simulink model "DA40_Flight_Model"  (R2023a)
settings: Solver=FixedStepAuto  StartTime=DCAM.startTime  StopTime=DCAM.endTime  FixedStep=DCAM.timeStep  RelTol=1e-3
undefined symbols (not defined in the file or in its folder): DCAM, Earth, WGS84
libraries: simulink x27, slpidlib x15, simulink_extras x6, sharedtransform x4, aerolibtransform2 x4, aerolibatmos2 x3, uavalgslib x2, aerolibwind2 x1
(part 6 of 6)

== matlab function DA40_Flight_Model/Correlator Simulation/Subsystem1/Generating GPS and Satellite Measurements1/Truth Model/Navigation1/Flight Mechanics and Systems Models/Engine + Prop Model/Subsystem/MATLAB Function ==
  data: X input; Aircraft_Airspeed output
function Aircraft_Airspeed = Calc_AC_Speed(X)
Aircraft_Airspeed = norm(X(1:3));
end

== matlab function DA40_Flight_Model/Correlator Simulation/Subsystem1/Generating GPS and Satellite Measurements1/Truth Model/Navigation1/Flight Mechanics and Systems Models/Engine + Prop Model/Subsystem/Manifold Pressure Calculation ==
  data: throttle input; Patm_inHg input; N input; Pman_inHg output; throttle output; Patm_inHg output
function [Pman_inHg,throttle,Patm_inHg]  = fcn(throttle,Patm_inHg,N)

Pman_inHg = Patm_inHg + (0.007*throttle - 0.0086)*N;

end

== matlab function DA40_Flight_Model/Correlator Simulation/Subsystem1/Generating GPS and Satellite Measurements1/Truth Model/Navigation1/Flight Mechanics and Systems Models/Engine + Prop Model/Subsystem/Propeller Dynamics ==
  data: V input; power input; Q_drive input size=1; Prop_Pitch input; rho input; n input; T output; Q output; eta_p output size=1; dOmega_dt output
function [T,Q,eta_p,dOmega_dt] = VarP_PropDynamics(V,power, Q_drive,Prop_Pitch,rho,n)

T = 0;
Q = 0;
eta_p = 0;
dOmega_dt = 0;

coder.extrinsic('griddedInterpolant')
coder.extrinsic('CTCQPropeff')

[T,Q,eta_p,dOmega_dt] = CTCQPropeff(Prop_Pitch,power,Q_drive,rho,V,n,[]);

end

== matlab function DA40_Flight_Model/Extended Kalman Filter/ECEF to BODY/MATLAB Function1 ==
  data: x output; pos input; y output; vel input; clk input; clkBias input; DCM_BL input; z output; u output; v output; w output; clk output; clkBias output; refLL input
function [x,y,z,u,v,w,clk,clkBias] = EarthToBodyStates(pos,vel,clk,clkBias,DCM_BL,refLL)
x = 0;
y = 0;
z = 0;
u = 0;
v = 0;
w = 0;

coder.extrinsic("EarthToBodyStates")

[x,y,z,u,v,w,clk,clkBias] = BodyToEarthStates(pos,vel,clk,clkBias,DCM_BL,refLL);

end

== matlab function DA40_Flight_Model/Correlator Simulation/Subsystem1/Generating GPS and Satellite Measurements1/Truth Model/Navigation1/Flight Mechanics and Systems Models/Gear/  ==
  data: U input; X input; mu input; Ground_Forces output; Ground_Moments output
function [Ground_Forces,Ground_Moments] = LDG_Model(U,X,mu)
%% Ground Contact points taken from powerpoint
Front_LDG = [1.634;0;0.983]';
Right_MG = [-0.5;1.447;0.893]';
Left_MG = [-0.5;-1.447;0.893]';
Prop_Strike = [2.379;0;0.847]';
Right_Wing = [0;5.53;-0.087]';
Left_Wing = [0;-5.53;-0.087]';
Tail_Strike = [-4.552;0;0.271]';
GC = [Front_LDG;Right_MG;Left_MG;Prop_Strike;Right_Wing;Left_Wing;Tail_Strike];
%% Spring and Damper Coeffs
k_r = 80000;
c_r = 14300;

k_f = 50000;
c_f = 11300;

k_b = 280000;
c_b = 26800;
%% Defining State Vector to make the coding easier
u = X(1);
v = X(2);
w = X(3);
p = X(4);
q = X(5);
r = X(6);
x = X(7);
y = X(8);
z = X(9);
phi = X(10);
theta = X(11);
psi = X(12);

ALTdot = -w;
ALT = -z;
%% State Derivatives
phidot = p + q*sin(phi)*tan(theta) + r*cos(phi)*tan(theta);
thetadot = q*cos(phi) - r*sin(phi);
%% Controls from Pilot
Brake_Setting = (U(1) + U(2))/2;
Steering_Control = U(3);
%% Friction while plane is in motion
Rolling_Friction = mu(1);
%% Calculations
%% Have to calculate each components distance from the ground...
del_S = zeros(7,1);
del_S_dot = zeros(7,1);
F = zeros(7,3);

del_S(1) = ALT + Front_LDG(1)*sin(theta) - Front_LDG(2)*sin(phi)*cos(theta) - Front_LDG(3)*cos(phi)*cos(theta);
del_S(2) = ALT + Right_MG(1)*sin(theta) - Right_MG(2)*sin(phi)*cos(theta) - Right_MG(3)*cos(phi)*cos(theta);
del_S(3) = ALT + Left_MG(1)*sin(theta) - Left_MG(2)*sin(phi)*cos(theta) - Left_MG(3)*cos(phi)*cos(theta);
del_S(4) = ALT + Prop_Strike(1)*sin(theta) - Prop_Strike(2)*sin(phi)*cos(theta) - Prop_Strike(3)*cos(phi)*cos(theta);
del_S(5) = ALT + Right_Wing(1)*sin(theta) - Right_Wing(2)*sin(phi)*cos(theta) - Right_Wing(3)*cos(phi)*cos(theta);
del_S(6) = ALT + Left_Wing(1)*sin(theta) - Left_Wing(2)*sin(phi)*cos(theta) - Left_Wing(3)*cos(phi)*cos(theta);
del_S(7) = ALT + Tail_Strike(1)*sin(theta) - Tail_Strike(2)*sin(phi)*cos(theta) - Tail_Strike(3)*cos(phi)*cos(theta);

%deltaS order
% 1 Nose Gear
% 2 Right Main Gear
% 3 Left Main Gear
% 4 Prop Strike
% 5 Right Wingtip
% 6 Left Wingtip
% 7 Tail Strike

del_S_dot(1) = ALTdot + Front_LDG(1)*cos(theta)*thetadot + Front_LDG(2)*(thetadot*sin(phi)*sin(theta) - phidot*cos(phi)*cos(theta)) + Front_LDG(3)*(thetadot*sin(theta)*cos(phi) + phidot*sin(theta)*sin(phi))+ del_S(1)*(cos(phi)*sin(theta)*thetadot + sin(phi)*cos(theta)*phidot);
if del_S(1) < 0
    F(1,3) = k_f*del_S(1) + c_f*del_S_dot(1);
else
    F(1,3) = 0;
end
del_S_dot(2) = ALTdot + Right_MG(1)*cos(theta)*thetadot + Right_MG(2)*(thetadot*sin(phi)*sin(theta) - phidot*cos(phi)*cos(theta)) + Right_MG(3)*(thetadot*sin(theta)*cos(phi) + phidot*sin(theta)*sin(phi))+ del_S(2)*(cos(phi)*sin(theta)*thetadot + sin(phi)*cos(theta)*phidot);
if del_S(2) < 0
    F(2,3) = k_r*del_S(2) + c_r*del_S_dot(2);
else
    F(2,3) = 0;
end
del_S_dot(3) = ALTdot + Left_MG(1)*cos(theta)*thetadot + Left_MG(2)*(thetadot*sin(phi)*sin(theta) - phidot*cos(phi)*cos(theta)) + Left_MG(3)*(thetadot*sin(theta)*cos(phi) + phidot*sin(theta)*sin(phi))+ del_S(3)*(cos(phi)*sin(theta)*thetadot + sin(phi)*cos(theta)*phidot);
if del_S(3) < 0
    F(3,3) = k_r*del_S(3) + c_r*del_S_dot(3);
else
    F(3,3) = 0;
end
del_S_dot(4) = ALTdot + Prop_Strike(1)*cos(theta)*thetadot + Prop_Strike(2)*(thetadot*sin(phi)*sin(theta) - phidot*cos(phi)*cos(theta)) + Prop_Strike(3)*(thetadot*sin(theta)*cos(phi) + phidot*sin(theta)*sin(phi));
if del_S(4) < 0
    F(4,3) = k_b*del_S(4) + c_b*del_S_dot(4);
else
    F(4,3) = 0;
end
del_S_dot(5) = ALTdot + Right_Wing(1)*cos(theta)*thetadot + Right_Wing(2)*(thetadot*sin(phi)*sin(theta) - phidot*cos(phi)*cos(theta)) + Right_Wing(3)*(thetadot*sin(theta)*cos(phi) + phidot*sin(theta)*sin(phi));
if del_S(5) < 0
    F(5,3) = k_b*del_S(5) + c_b*del_S_dot(5);
else
    F(5,3) = 0;
end
del_S_dot(6) = ALTdot + Left_Wing(1)*cos(theta)*thetadot + Left_Wing(2)*(thetadot*sin(phi)*sin(theta) - phidot*cos(phi)*cos(theta))+ Left_Wing(3)*(thetadot*sin(theta)*cos(phi) + phidot*sin(theta)*sin(phi));
if del_S(6) < 0
    F(6,3) = k_b*del_S(6) + c_b*del_S_dot(6);
else
    F(6,3) = 0;
end

del_S_dot(7) = ALTdot + Tail_Strike(1)*cos(theta)*thetadot + Tail_Strike(2)*(thetadot*sin(phi)*sin(theta) - phidot*cos(phi)*cos(theta)) + Tail_Strike(3)*(thetadot*sin(theta)*cos(phi) + phidot*sin(theta)*sin(phi));
if del_S(7) < 0
    F(7,3) = k_b*del_S(7) + c_b*del_S_dot(7);
else
    F(7,3) = 0;
end
%% Calculating the velo seen by the LDG

VxB = u - r.*GC(:,2) + q.*(GC(:,3) + del_S);
VyB = v + r.*GC(:,1) - p.*(GC(:,3) + del_S);
VzB = w - q.*GC(:,1) + p.*GC(:,2);

Vxge = cos(theta).*VxB + (sin(phi).*sin(theta)).*VyB + (cos(phi)*sin(theta)).*VzB;
Vyge = cos(phi).*VyB + (-sin(phi)).*VzB;

Steering_Control = [Steering_Control,0,0,0,0,0,0]';
uk  = VxB.*cos(Steering_Control) + VyB.*sin(Steering_Control);

mu_s = 0.8;
C_p = 1.1;
B_p = 7;
mu_br = 0.7*Brake_Setting;
mu_rb = zeros(3,1);
mu_Y = zeros(3,1);
for i = 1:3
    if abs(uk(i)) < 1e-4
        mu_rb(i) = 0;
    else
        mu_rb(i) =  (Rolling_Friction + mu_br).*sign(uk(i));
    end
    
    mu_y_max = sqrt(mu_s^2 - mu_rb(i)^2);
    Sy =  Steering_Control(i) - atan(Vyge(i)/(Vxge(i) + 0.00000001 ));
    if abs(uk(i)) < 0.001
        mu_Y(i) = 0;
    else
        mu_Y(i) = -mu_y_max*sin(C_p*atan(B_p.*Sy));
    end
end
%% Calculating the x and y forces...
F(1:3,1) = mu_rb.*F(1:3,3);
F(1:3,2) = mu_Y.*F(1:3,3);
%% Converting to Body-Fixed Axis to output...
F_B = zeros(7,3);
F_B(:,1) = cos(theta).*cos(-Steering_Control).*F(:,1) + cos(theta).*F(:,2) - sin(theta).*F(:,3);
F_B(:,2)= (sin(phi).*sin(theta).*cos(-Steering_Control)-cos(phi).*sin(-Steering_Control)).*F(:,1) + (sin(phi).*sin(theta).*sin(-Steering_Control) + cos(phi).*cos(-Steering_Control)).*F(:,2) + sin(phi).*cos(theta).*F(:,3);
F_B(:,3) = (cos(phi).*sin(theta).*cos(-Steering_Control) + sin(phi).*sin(-Steering_Control)).*F(:,1) + (cos(phi).*sin(theta).*sin(-Steering_Control)-sin(phi).*cos(-Steering_Control)).*F(:,2) + (cos(phi).*cos(theta)).*F(:,3);

NG_Mom = cross(Front_LDG,F(1,:));
RMG_Mom = cross(Right_MG, F(2,:));
LMG_Mom = cross(Left_MG, F(3,:));
Prop_Strike_Mom = cross(Prop_Strike,F(4,:));
RWT_Mom = cross(Right_Wing,F(5,:));
LWT_Mom = cross(Left_Wing,F(6,:));
Tail_Strike_Mom = cross(Tail_Strike, F(7,:));

Ground_Forces = [sum(F_B(:,1)),sum(F_B(:,2)),sum(F_B(:,3))];
Ground_Moments = (NG_Mom + RMG_Mom + LMG_Mom + Prop_Strike_Mom + RWT_Mom + LWT_Mom + Tail_Strike_Mom);
end

== matlab function DA40_Flight_Model/Correlator Simulation/Subsystem1/Generating GPS and Satellite Measurements1/Truth Model/Navigation1/Flight Mechanics and Systems Models/Gravity/MATLAB Function ==
  data: X input; F_grav_b output; Mass_Properties input; CG input; M_grav_b output
function [F_grav_b,M_grav_b] = Grav_Forces(X,Mass_Properties,CG)
%% Defining State Vector to Code Easier
u = X(1);
v = X(2);
w = X(3);
p = X(4);
q = X(5);
r = X(6);
x = X(7);
y = X(8);
z = X(9);
phi = X(10);
theta = X(11);
psi = X(12);

g = 9.81;

F_grav_b = Mass_Properties.*[-g*sin(theta);g*sin(phi)*cos(theta);g*cos(phi)*cos(theta)];

M_grav_b = cross(CG,F_grav_b);

== matlab function DA40_Flight_Model/Correlator Simulation/Subsystem1/Generating GPS and Satellite Measurements1/Truth Model/Navigation1/Flight Mechanics and Systems Models/Strip Theory Aero + Propulsive Forces/Strip_Theory_Modeling ==
  data: atmos input; X input; U input; stripGeom input; Strip_Theory_Forces output; Strip_Theory_Moments output
function [Strip_Theory_Forces,Strip_Theory_Moments] = Strip_Theory(atmos,X,U,stripGeom)
Strip_Theory_Forces = [0;0;0];
Strip_Theory_Moments = [0;0;0];

coder.extrinsic('griddedInterpolant')
coder.extrinsic('AC_Strip_Theory')

[Strip_Theory_Forces,Strip_Theory_Moments] = AC_Strip_Theory(atmos(4),X,U,stripGeom);

== matlab function DA40_Flight_Model/Correlator Simulation/Subsystem1/Subsystem2/Generating PSR//Carrier Frequency Measurements1/MATLAB Function ==
  data: usrX input; usrY input; usrZ input; clk input; pseudoranges output; satX input; satY input; satZ input; unitVectors output
function [pseudoranges,unitVectors] = calcPSR(usrX,usrY,usrZ,clk,satX,satY,satZ)

dx2 = (usrX - satX).^2;
dy2 = (usrY - satY).^2;
dz2 = (usrZ - satZ).^2;

r = sqrt(dx2 + dy2 + dz2);
pseudoranges =  r + clk;

ux = (usrX - satX)./r;
uy = (usrY - satY)./r;
uz = (usrZ - satZ)./r;

unitVectors = [ux;uy;uz];

end

== matlab function DA40_Flight_Model/Correlator Simulation/Subsystem1/Subsystem2/Generating PSR//Carrier Frequency Measurements1/MATLAB Function1 ==
  data: unitVectors input; carrFrequency output; usrU input; usrV input; usrW input; satU input; satV input; satW input; clkDrift input; L1Freq input; IFFreq input
function carrFrequency = calcCarrFreq(unitVectors,usrU,usrV,usrW,satU,satV,satW,clkDrift,L1Freq,IFFreq)

satVel = [satU;satV;satW];
usrVel = [usrU;usrV;usrW];

velLOS = unitVectors.*(satVel - usrVel);
carrFrequency = (1 - velLOS/c)*L1Freq / (1 + clkDrift/c) - L1Freq + IFFreq;

end

== matlab function DA40_Flight_Model/Correlator Simulation/Subsystem1/Subsystem2/Subsystem2/MATLAB Function1 ==
  data: svClockBias input; dSvClk output; initialSVClockBias input
function dSvClk = calculateClockDifference(svClockBias,initialSVClockBias)

dSvClk = svClockBias - initialSVClockBias;

end

== matlab function DA40_Flight_Model/Correlator Simulation/Subsystem1/Subsystem2/Subsystem2/MATLAB Function2 ==
  data: doppler input; estimatedCodeFrequency output; chiprate input; L1freq input
function estimatedCodeFrequency = fcn(doppler,chiprate,L1freq)

estimatedCodeFrequency = doppler + chiprate/L1freq + chiprate;

== matlab function DA40_Flight_Model/Correlator Simulation/Subsystem1/Subsystem2/Subsystem2/MATLAB Function3 ==
  data: initialDoppler input; initialCodeFrequency output; initialChiprate input; L1freq input
function initialCodeFrequency = fcn(initialDoppler,initialChiprate,L1freq)

initialCodeFrequency = initialDoppler + initialChiprate/L1freq + initialChiprate;

== matlab function DA40_Flight_Model/Correlator Simulation/Subsystem1/Subsystem2/Subsystem2/Subsystem2/MATLAB Function1 ==
  data: samplesPerPDI input; initialCodeFrequency input; initialCodePhase input; codeChangePerSample output; measuredCodeFrequency input; initialCodePhase output; chipRate input; dSvClk input
function [codeChangePerSample,initialCodePhase]  = fcn(samplesPerPDI,initialCodeFrequency,initialCodePhase,measuredCodeFrequency,chipRate,dSvClk)

codeChangePerSample = (measuredCodeFrequency - initialCodeFrequency + dSvClk*chipRate)/samplesPerPDI;

initialCodePhase = initialCodePhase;

end

== matlab function DA40_Flight_Model/Correlator Simulation/Subsystem1/Subsystem2/Subsystem2/Subsystem2/MATLAB Function4 ==
  data: samplesPerPDI input; initialCarrierFrequency input; sampleVector output; carrierChangePerSample output; measuredCarrierFrequency input
function [sampleVector,carrierChangePerSample]  = fcn(samplesPerPDI,initialCarrierFrequency,measuredCarrierFrequency)

sampleVector = 0:samplesPerPDI;
carrierChangePerSample = (measuredCarrierFrequency - initialCarrierFrequency)/samplesPerPDI;

end

== matlab function DA40_Flight_Model/Correlator Simulation/Subsystem1/Subsystem2/Subsystem4/MATLAB Function1 ==
  data: sampleVector input; MeasuredCodeFrequency output; codeChangePerSample input; initialCodePhase input
function MeasuredCodeFrequency = calcMeasuredCodeFrequency(sampleVector,codeChangePerSample,initialCodePhase)

MeasuredCodeFrequency = sampleVector*codeChangePerSample + measuredCarrierFrequency;

trueCodePhase = sampleVec(idx)*codeChangePerSample + initialCodePhase;
trueCodePhase = trueCodePhaseVec(idx);

end

== matlab function DA40_Flight_Model/Correlator Simulation/Subsystem1/Subsystem2/Subsystem4/MATLAB Function3 ==
  data: sampleVector input; MeasuredCarrierFrequency output; carrierChangePerSample input; measuredCarrierFrequency input
function MeasuredCarrierFrequency = calcMeasuredCarrierFrequency(sampleVector,carrierChangePerSample,measuredCarrierFrequency)

MeasuredCarrierFrequency = sampleVector*carrierChangePerSample + measuredCarrierFrequency;

end

== matlab function DA40_Flight_Model/Correlator Simulation/MATLAB Function1 ==
  data: IE input; carrierFreqResiduals output; QE input; IP input; QP input; IL input; QL input; codeFreqResiduals output
function [carrierFreqResiduals,codeFreqResiduals] = calcDiscriminators(IE,QE,IP,QP,IL,QL)

carrierFreqResiduals = atan(QP/IP)/2/pi;
codeFreqResiduals = 1/4*((IE^2+QE^2) - (IL^2 + QL^2))/((IE^2+QE^2) + (IL^2 + QL^2));

== matlab function DA40_Flight_Model/Extended Kalman Filter/Body To ECEF/MATLAB Function ==
  data: DCM_BN input; DCM_BE output; DCM_NE input
function DCM_BE = fcn(DCM_BN,DCM_NE)

DCM_BE = DCM_NE*DCM_BN;

end

== matlab function DA40_Flight_Model/Correlator Simulation/Subsystem1/Generating GPS and Satellite Measurements/Truth Model/Environment/MATLAB Function ==
  data: windVectorNav input; windVectorBody output; states input
function windVectorBody = windRotation(windVectorNav,states)

DCMBN = genDCM('rad',[states(12),states(11),states(10)], [3 2 1]);

windVectorBody = DCMBN'*[windVectorNav; 0];

end
